simulink model "PD"  (Simulink 9.3)
settings: Solver=ode5  StartTime=0.0  StopTime=1000  FixedStep=0.1  RelTol=1e-3  EnableMultiTasking=on
undefined symbols (not defined in the file): sigbuilder_block
libraries: fuzblock x1
settings Model: Creator=lemin  LastModifiedBy=forev
settings DataIOCC: LimitDataPoints=on
settings OptimizationCC: ExpressionDepthLimit=2147483647
settings DebuggingCC: SolverPrmCheckMsg=warning  StateNameClashWarn=warning  SFExecutionAtInitializationDiag=warning
settings GRTTargetCC: GeneratePreprocessorConditionals=Disable all

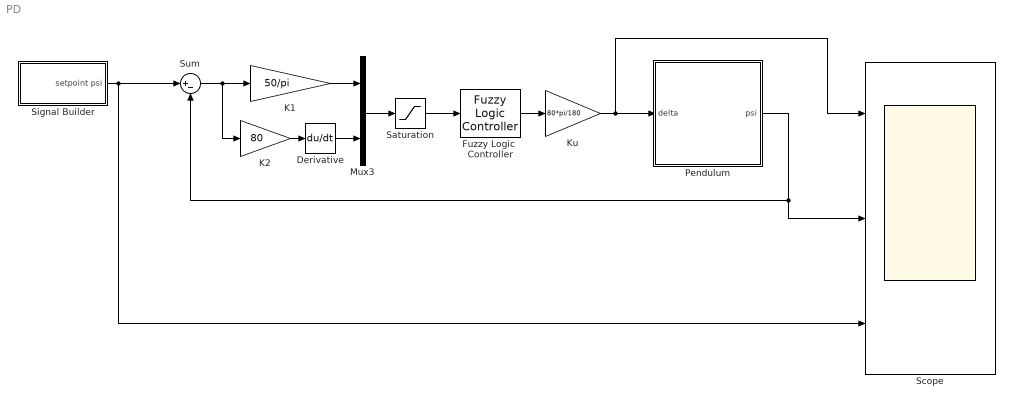
== system PD ==
  Derivative : Derivative
  Fuzzy Logic  Controller : fuzblock/Fuzzy Logic  Controller  FIS='PD-Ship.fis'  OutputSampleNumber=101  DataType=double  FuzzifiedInputs=off  RuleFiringStrengths=off  RuleOutputs=off  AggregatedOutputs=off  SimulateUsing=Interpreted execution  OutOfRangeInputValueMessage=warning  NoRuleFiredMessage=warning  EmptyOutputFuzzySetMessage=warning
  "K1 " : Gain  Gain=50/pi
  K2 : Gain  Gain=80
  Ku : Gain  Gain=80*pi/180
  Mux3 : Mux  Inputs=2
  Pendulum : Subsystem  mask{l=250, v=8, k=5.88*8/250, t1=-16.91*250/8, t2=0.45*250/8, t3=1.43*250/8, psi3dot0=0, psi2dot0=0, psi1dot0=0}
      mask prompts: l "chieu dai tau"; v "van toc tau"
  Saturation : Saturate  UpperLimit=1  LowerLimit=-1
  Scope : Scope  NumInputPorts=3
  Signal Builder : Subsystem  Tag=STV Subsys  LoadFcn=sigbuilder_block('load');  StartFcn=sigbuilder_block('start');  StopFcn=sigbuilder_block('stop');  ClipboardFcn=sigbuilder_block('clipboard');  mask(Sigbuilder block){tuvar=[0:10]}
      mask help: Simulink:masks:SigbuilderBlock_MD
      mask init:
      | if ~strcmp(get_param(bdroot(gcbh),'SimulationStatus'),'stopped') tuvar = sigbuilder_block('maskInit'); end
      settings: CopyFcn=sigbuilder_block('copy');  DeleteFcn=sigbuilder_block('delete');  ModelCloseFcn=sigbuilder_block('modelClose');  PreSaveFcn=sigbuilder_block('preSave');  PauseFcn=sigbuilder_block('pause');  ContinueFcn=sigbuilder_block('continue');  NameChangeFcn=sigbuilder_block('namechange');  OpenFcn=sigbuilder_block('open',[345.6 54.6 550.8 400.2 ]);  CloseFcn=sigbuilder_block('close');
      mask Display: plot(0, 0, 100, 100,[2, 2, 32, 32, 2], [68, 8, 8, 68, 68],[32, 2], [38, 38], [32, 19, 2],[53, 60, 44], [32, 17, 17, 2],[16, 16, 31, 31]);txt = getActiveGroup(gcbh);text(2, 100, txt,'verticalAlignment', 'top');
  Sum : Sum  Inputs=|+-
  wires:
  Fuzzy Logic  Controller/1 -> Ku/1
  Ku/1 -> Scope/1, Pendulum/1("delta ")
  Sum/1 -> K2/1, "K1 "/1
  K2/1 -> Derivative/1
  Derivative/1 -> Mux3/2
  "K1 "/1 -> Mux3/1
  Pendulum/1(psi) -> Scope/2, Sum/2
  Saturation/1 -> Fuzzy Logic  Controller/1
  Mux3/1 -> Saturation/1
  Signal Builder/1(setpoint psi) -> Scope/3, Sum/1

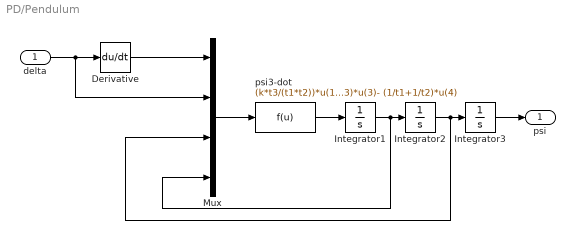
== system PD/Pendulum ==
  "delta " : Inport
  Derivative : Derivative
  Integrator1 : Integrator  InitialCondition=psi3dot0
  Integrator2 : Integrator  InitialCondition=psi2dot0
  Integrator3 : Integrator  InitialCondition=psi1dot0
  Mux : Mux
  psi3-dot : Fcn  Expr=(k*t3/(t1*t2))*u(1)+(k/(t1*t2))*u(2) - (1/(t1*t2))*u(3) - (1/(t1*t2))*u(3)*u(3)*u(3)- (1/t1+1/t2)*u(4)
  psi : Outport
  wires:
  "delta "/1 -> Mux/2, Derivative/1
  psi3-dot/1 -> Integrator1/1
  Derivative/1 -> Mux/1
  Mux/1 -> psi3-dot/1
  Integrator1/1 -> Mux/4, Integrator2/1
  Integrator2/1 -> Mux/3, Integrator3/1
  Integrator3/1 -> psi/1

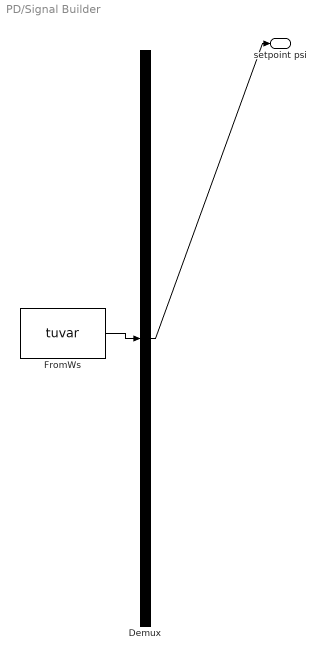
== system PD/Signal Builder ==
  Demux : Demux  Tag=STV Demux  Outputs=1
  FromWs : FromWorkspace  Tag=STV FromWs  VariableName=tuvar  SampleTime=0  SigBuilderData=DataTag0  VnvData=DataTag1
      SigBuilderData=|
      | common.afterFinalStr = 'Extrapolate'
      | common.sampleTime = 0
      | dataSet.timeRange = [0 1000]
      | dataSet.name = 'Group 1'
      | sbobj.Groups.Name = 'Group 1'
      | sbobj.Groups.Signals.Name = 'setpoint psi'
      | sbobj.Groups.Signals.XData = [0 332 332 1000]
      | sbobj.Groups.Signals.YData = [0 0 0.445 0.445]
      | sbobj.Groups.TimeRange = [0 1000]
  setpoint psi : Outport  Tag=STV Outport
  wires:
  FromWs/1 -> Demux/1
  Demux/1 -> setpoint psi/1
